simulink model "chart_simulink_2015"  (R2015a)
settings: Solver=ode45  StartTime=0.0  StopTime=10.0  RelTol=1e-3
settings Model: Creator=Administrator  LastModifiedBy=Administrator

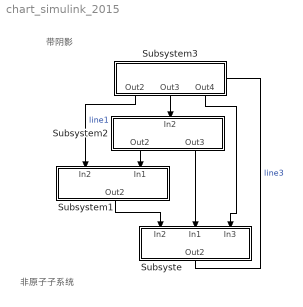
== system chart_simulink_2015 ==
  note: 带阴影
  note: 非原子子系统
  Subsyste : Subsystem
      mask Display: disp('no shadow\nnot atomic unit')
  Subsystem1 : Subsystem  TreatAsAtomicUnit=on
      mask Display: disp('no shadow\natomic unit')
  Subsystem2 : Subsystem
      mask Display: disp('带阴影\n非原子子系统')
  Subsystem3 : Subsystem  TreatAsAtomicUnit=on
      settings: AttributesFormatString=子系统注释
      mask Display: disp('带阴影\n原子子系统')
  wires:
  Subsyste/1(Out2) -> Subsystem3/Enable  "line3"
  Subsystem3/2(Out3) -> Subsystem2/1(In2)
  Subsystem3/1(Out2) -> Subsystem1/1(In2)  "line1"
  Subsystem2/1(Out2) -> Subsystem1/2(In1)
  Subsystem3/3(Out4) -> Subsyste/3(In3)
  Subsystem2/2(Out3) -> Subsyste/2(In1)
  Subsystem1/1(Out2) -> Subsyste/1(In2)

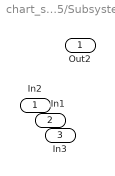
== system chart_simulink_2015/Subsyste ==
  In2 : Inport
  In1 : Inport  Port=2
  In3 : Inport  Port=3
  Out2 : Outport

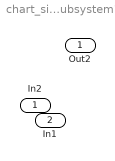
== system chart_simulink_2015/Subsystem1 ==
  In2 : Inport
  In1 : Inport  Port=2
  Out2 : Outport

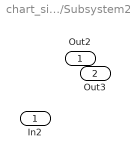
== system chart_simulink_2015/Subsystem2 ==
  In2 : Inport
  Out2 : Outport
  Out3 : Outport  Port=2

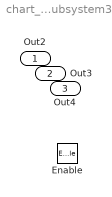
== system chart_simulink_2015/Subsystem3 ==
  Enable : EnablePort
  Out2 : Outport
  Out3 : Outport  Port=2
  Out4 : Outport  Port=3
